simulink model "testforexam"  (R2016b)
settings: Solver=VariableStepAuto  StartTime=0.0  StopTime=100.0  RelTol=1e-3
settings Model: Creator=ASUS  LastModifiedBy=ASUS

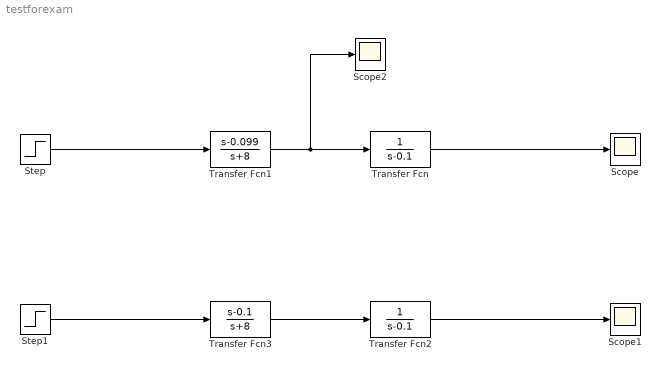
== system testforexam ==
  Scope : Scope
  Scope1 : Scope
  Scope2 : Scope
  Step : Step  SampleTime=0
  Step1 : Step  SampleTime=0
  Transfer Fcn : TransferFcn  Denominator=[1 -0.1]
  Transfer Fcn1 : TransferFcn  Numerator=[1 -0.099]  Denominator=[1 8]
  Transfer Fcn2 : TransferFcn  Denominator=[1 -0.1]
  Transfer Fcn3 : TransferFcn  Numerator=[1 -0.1]  Denominator=[1 8]
  wires:
  Transfer Fcn1/1 -> Scope2/1, Transfer Fcn/1
  Transfer Fcn/1 -> Scope/1
  Step/1 -> Transfer Fcn1/1
  Transfer Fcn3/1 -> Transfer Fcn2/1
  Transfer Fcn2/1 -> Scope1/1
  Step1/1 -> Transfer Fcn3/1
